simulink model "motor_position_control"  (Simulink 9.1)
settings: Solver=ode45  StartTime=0.0  StopTime=10.0  RelTol=1e-3  EnableMultiTasking=on
settings Model: SuppressorTable=22 serialization::archive 11 0 6 0 0 0 0 0  Creator=arturogilaparicio  LastModifiedBy=arturogilaparicio
settings DataIOCC: LimitDataPoints=on
settings DebuggingCC: UnderspecifiedInitializationDetection=Simplified  MergeDetectMultiDrivingBlocksExec=error
settings GRTTargetCC: GeneratePreprocessorConditionals=Disable all  CombineOutputUpdateFcns=on  GRTInterface=off

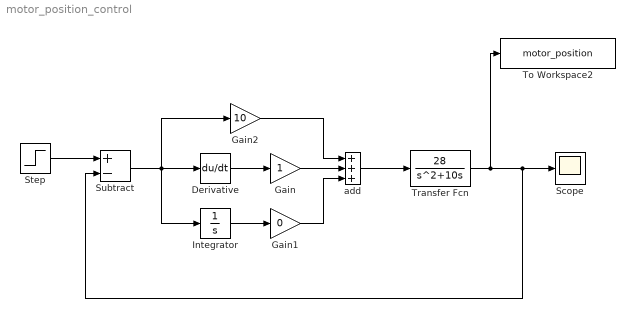
== system motor_position_control ==
  Derivative : Derivative
  Gain : Gain
  Gain1 : Gain  Gain=0
  Gain2 : Gain  Gain=10
  Integrator : Integrator
  Scope : Scope
  Step : Step  Time=0  After=5  SampleTime=0
  Subtract : Sum  Inputs=+-
  To Workspace2 : ToWorkspace  VariableName=motor_position  SampleTime=-1
  Transfer Fcn : TransferFcn  Numerator=[28]  Denominator=[1 10 0]
  add : Sum  Inputs=+++
  wires:
  add/1 -> Transfer Fcn/1
  Gain/1 -> add/2
  Gain2/1 -> add/1
  Gain1/1 -> add/3
  Derivative/1 -> Gain/1
  Integrator/1 -> Gain1/1
  Subtract/1 -> Integrator/1, Gain2/1, Derivative/1
  Step/1 -> Subtract/1
  Transfer Fcn/1 -> To Workspace2/1, Scope/1, Subtract/2
